simulink model "xiti4_12Sine"  (Simulink 5.0)
settings: Solver=ode45  SolverMode=SingleTasking  StartTime=0.0  StopTime=80  FixedStep=0.25  RelTol=1e-3
values from neighbouring files (symbols this model uses):
  kd = kp*pi/(4*wr)    [xiti4_13Dm.m]    (also in xiti4_13Dm1.m)
  ki = kp*wr/pi    [xiti4_13Dm.m]    (also in xiti4_13Dm1.m)
  kp = 0.6*kr    [xiti4_13Dm.m]    (also in xiti4_13Dm1.m)
libraries: simulink x1
settings Model: LastModifiedBy=ThinkPad  ExtModeTrigMode=oneshot  ExtModeArmWhenConnect=off  LimitDataPoints=off  BooleanDataType=off

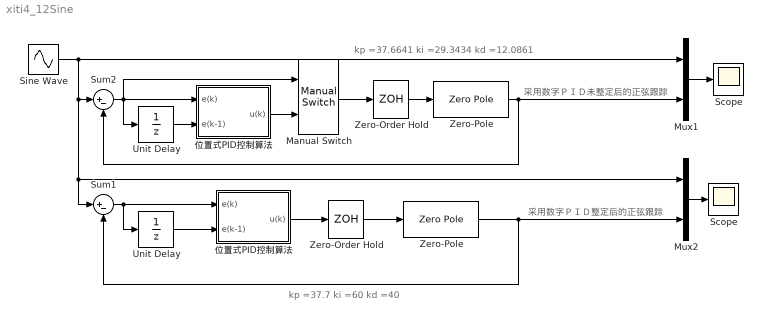
== system xiti4_12Sine ==
  note: 采用数字ＰＩＤ未整定后的正弦跟踪
  note: kp =37.6641 ki =29.3434 kd =12.0861
  note: 采用数字ＰＩＤ整定后的正弦跟踪
  note: kp =37.7 ki =60 kd =40
  " Scope" : Scope
      settings: YMin=-3.5  YMax=1  MaxDataPoints=500000
  "Manual Switch " : simulink/Signal Routing/Manual Switch  sw=0  action=0
  Mux1 : Mux  Inputs=2
  Mux2 : Mux  Inputs=2
  "Scope " : Scope
      settings: YMin=-3.5  YMax=1  MaxDataPoints=500000
  Sine Wave : Sin  Amplitude=0.5  Frequency=0.05*pi  SampleTime=0
  Sum1 : Sum  Inputs=|+-  SaturateOnIntegerOverflow=on
  Sum2 : Sum  Inputs=|+-  SaturateOnIntegerOverflow=on
  Unit Delay : UnitDelay  SampleTime=0.25
  "Unit Delay " : UnitDelay  SampleTime=0.25
  Zero-Order Hold : ZeroOrderHold  SampleTime=0.25
  "Zero-Order Hold " : ZeroOrderHold  SampleTime=0.25
  Zero-Pole : ZeroPole  Zeros=[]  Poles=[-0.5 -0.2]  Gain=[0.1]
  "Zero-Pole " : ZeroPole  Zeros=[]  Poles=[-0.5 -0.2]  Gain=[0.1]
  "位置式PID控制算法 " : Subsystem
  "位置式PID控制算法  " : Subsystem
  wires:
  Sine Wave/1 -> Mux1/1, Sum2/1, Sum1/1, Mux2/1
  Mux1/1 -> "Scope "/1
  Zero-Pole/1 -> Mux1/2, Sum2/2
  "Unit Delay "/1 -> "位置式PID控制算法 "/2(e(k-1))
  Sum2/1 -> "Manual Switch "/1, "Unit Delay "/1, "位置式PID控制算法 "/1(e(k))
  "位置式PID控制算法 "/1(u(k)) -> "Manual Switch "/2
  "Zero-Order Hold "/1 -> Zero-Pole/1
  "Manual Switch "/1 -> "Zero-Order Hold "/1
  Mux2/1 -> " Scope"/1
  "Zero-Pole "/1 -> Mux2/2, Sum1/2
  Unit Delay/1 -> "位置式PID控制算法  "/2(e(k-1))
  Sum1/1 -> "位置式PID控制算法  "/1(e(k)), Unit Delay/1
  "位置式PID控制算法  "/1(u(k)) -> Zero-Order Hold/1
  Zero-Order Hold/1 -> "Zero-Pole "/1

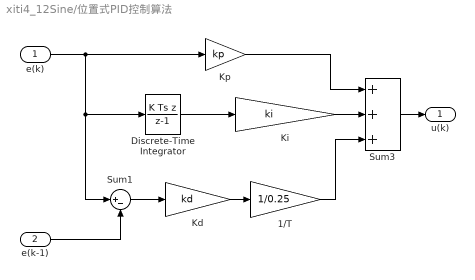
== system xiti4_12Sine/位置式PID控制算法  ==
  e(k) : Inport
  e(k-1) : Inport  Port=2
  1/T : Gain  Gain=1/0.25  SaturateOnIntegerOverflow=on
  Discrete-Time Integrator : DiscreteIntegrator  IntegratorMethod=Backward Euler  SampleTime=0.25
  Kd : Gain  Gain=kd  SaturateOnIntegerOverflow=on
  Ki : Gain  Gain=ki  SaturateOnIntegerOverflow=on
  Kp : Gain  Gain=kp  SaturateOnIntegerOverflow=on
  Sum1 : Sum  Inputs=|+-  SaturateOnIntegerOverflow=on
  Sum3 : Sum  Inputs=+++  SaturateOnIntegerOverflow=on
  u(k) : Outport
  wires:
  e(k-1)/1 -> Sum1/2
  1/T/1 -> Sum3/3
  Kd/1 -> 1/T/1
  Sum3/1 -> u(k)/1
  Ki/1 -> Sum3/2
  Kp/1 -> Sum3/1
  e(k)/1 -> Sum1/1, Discrete-Time Integrator/1, Kp/1
  Sum1/1 -> Kd/1
  Discrete-Time Integrator/1 -> Ki/1

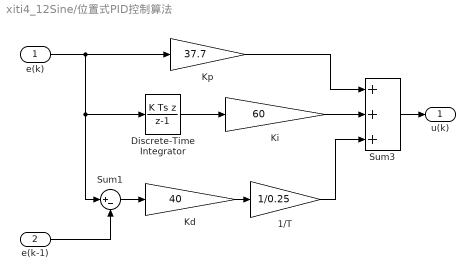
== system xiti4_12Sine/位置式PID控制算法   ==
  e(k) : Inport
  e(k-1) : Inport  Port=2
  1/T : Gain  Gain=1/0.25  SaturateOnIntegerOverflow=on
  Discrete-Time Integrator : DiscreteIntegrator  IntegratorMethod=Backward Euler  SampleTime=0.25
  Kd : Gain  Gain=40  SaturateOnIntegerOverflow=on
  Ki : Gain  Gain=60  SaturateOnIntegerOverflow=on
  Kp : Gain  Gain=37.7  SaturateOnIntegerOverflow=on
  Sum1 : Sum  Inputs=|+-  SaturateOnIntegerOverflow=on
  Sum3 : Sum  Inputs=+++  SaturateOnIntegerOverflow=on
  u(k) : Outport
  wires:
  Discrete-Time Integrator/1 -> Ki/1
  Sum1/1 -> Kd/1
  e(k)/1 -> Kp/1, Discrete-Time Integrator/1, Sum1/1
  Kp/1 -> Sum3/1
  Ki/1 -> Sum3/2
  Sum3/1 -> u(k)/1
  Kd/1 -> 1/T/1
  1/T/1 -> Sum3/3
  e(k-1)/1 -> Sum1/2
